simulink model "force_control"  (R2021b)
settings: Solver=FixedStepAuto  StartTime=0.0  StopTime=5  FixedStep=Ts  RelTol=1e-3
undefined symbols (not defined in the file): dqi, fd, invMd, K, KD, KF, KI, KP, Md, myRobot, qf, qi, qr, xr
libraries: vrlib x1
settings Model: Creator=simon  LastModifiedBy=luigi
settings SolverCC: ZeroCrossControl=DisableAll  AlgebraicLoopSolver=TrustRegion
settings DebuggingCC: SFMachineParentedDataDiag=warning

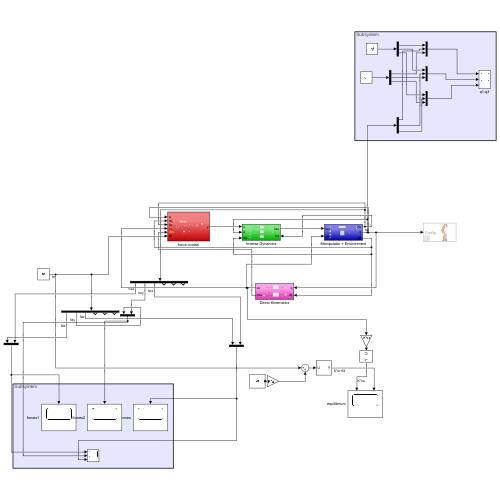
[thumbnail: Simulink's stored preview of the top-level diagram]
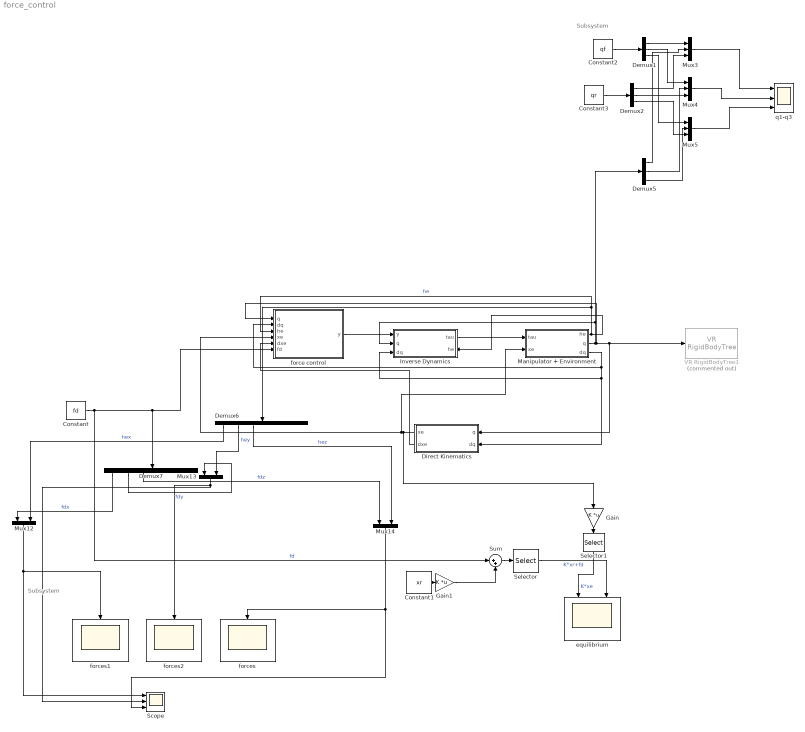
== system force_control ==
  note: Subsystem
  note: Subsystem
  Constant : Constant  Value=fd
  Constant1 : Constant  Value=xr
  Constant2 : Constant  Value=qf
  Constant3 : Constant  Value=qr
  Demux1 : Demux  Outputs=3
  Demux2 : Demux  Outputs=3
  Demux5 : Demux  Outputs=myRobot.N
  Demux6 : Demux  Outputs=6
  Demux7 : Demux  Outputs=6
  Direct Kinematics : Subsystem
  Gain : Gain  Gain=K  Multiplication=Matrix(K*u)
  Gain1 : Gain  Gain=K  Multiplication=Matrix(K*u)
  Inverse Dynamics : Subsystem
      settings: PortSchema="{\"entries\":[{\"content\":{\"sides\":[{\"content\":{\"connectorIds\":[\"In1\",\"In2\",\"In3\"]},\"type\":\"ConnectorPlacement.EquallySpacedRectSide\",\"uuid\":\"75fd2aef-6636-4229-8361-fd4aaeafc71d\"},{\"content\":{\"connectorIds\":[\"Out1\",\"In4\"],\"side\":\"RIGHT\"},\"type\":\"ConnectorPlacement.EquallySpacedRectSide\",\"uuid\":\"1144ef1f-b296-4ded-9ece-76b41f9ae70a\"},{\"content\":{\"connectorIds\":[],\"side\":\"TOP\"},\"type\":\"ConnectorPlacement.EquallySpacedRectSide\",\"uuid\":\"a2369661-a37d-42fa-931f-950a2098898d\"},{\"content\":{\"connectorIds\":[],\"side\":\"BOTTOM\"},\"type\":\"ConnectorPlacement.EquallySpacedRectSide\",\"uuid\":\"99474d0a-a266-4b98-966c-e86b0204795e\"},{\"content\":{\"connectorIds\":[],\"side\":\"HIDDEN\"},\"type\":\"ConnectorPlacement.EquallySpacedRectSide\",\"uuid\":\"b2ea56db-8612-481b-8b10-64691d881ee0\"}]},\"type\":\"ConnectorPlacement.EquallySpacedConnector\",\"uuid\":\"7eb160dc-bfe8-4791-8ee2-e581093abb5e\"}],\"packageUris\":[\"http://schema.mathworks.com/mf0/Connector/R2020b\"],\"version\":\"1.0\"}"
  Manipulator + Environment : Subsystem
  Mux12 : Mux  Inputs=2
  Mux13 : Mux  Inputs=2
  Mux14 : Mux  Inputs=2
  Mux3 : Mux  Inputs=3
  Mux4 : Mux  Inputs=3
  Mux5 : Mux  Inputs=3
  Scope : Scope  NumInputPorts=3
  Selector : Selector  InputPortWidth=6  IndexOptions=Index vector (dialog)  Indices=3  OutputSizes=1
  Selector1 : Selector  InputPortWidth=6  IndexOptions=Index vector (dialog)  Indices=3  OutputSizes=1
  Sum : Sum  Inputs=|++
  VR RigidBodyTree1 : vrlib/VR RigidBodyTree  Commented=on  RBT=rbt  useRBT=on  Ts=-1  ForceViewerOpen=on
      settings: SourceProductBaseCode=SL
  equilibrium : Scope  NumInputPorts=2
  force control : Subsystem
  forces : Scope
  forces1 : Scope
  forces2 : Scope
  q1-q3 : Scope  NumInputPorts=3
  wires:
  Direct Kinematics/2(dxe) -> force control/5(dxe)
  force control/1(y) -> Inverse Dynamics/1(y)
  Inverse Dynamics/1(tau) -> Manipulator + Environment/1(tau)
  Manipulator + Environment/3(dq) -> Inverse Dynamics/3(dq), Direct Kinematics/2(dq), force control/2(dq)
  Manipulator + Environment/1(he) -> Demux6/1, force control/3(he), Inverse Dynamics/4(he)  "he"
  Demux7/3 -> Mux14/1  "fdz"
  Direct Kinematics/1(xe) -> Manipulator + Environment/2(xe), force control/4(xe), Gain/1
  Constant/1 -> force control/6(fd), Demux7/1, Sum/1  "fd"
  Demux7/2 -> Mux13/1  "fdy"
  Demux7/1 -> Mux12/1  "fdx"
  Demux6/2 -> Mux13/2  "hey"
  Demux6/1 -> Mux12/2  "hex"
  Demux6/3 -> Mux14/2  "hez"
  Constant1/1 -> Gain1/1
  Selector1/1 -> equilibrium/1  "K*xe"
  Gain/1 -> Selector1/1
  Gain1/1 -> Sum/2
  Sum/1 -> Selector/1
  Selector/1 -> equilibrium/2  "K*xr+fd"
  Mux13/1 -> Scope/2, forces2/1
  Mux14/1 -> Scope/3, forces/1
  Mux12/1 -> Scope/1, forces1/1
  Manipulator + Environment/2(q) -> VR RigidBodyTree1/1, Direct Kinematics/1(q), force control/1(q), Demux5/1, Inverse Dynamics/2(q)
  Demux2/3 -> Mux5/3
  Constant3/1 -> Demux2/1
  Demux2/1 -> Mux3/3
  Demux2/2 -> Mux4/3
  Mux4/1 -> q1-q3/2
  Constant2/1 -> Demux1/1
  Demux1/3 -> Mux5/1
  Mux3/1 -> q1-q3/1
  Demux5/2 -> Mux4/2
  Demux5/3 -> Mux5/2
  Mux5/1 -> q1-q3/3
  Demux5/1 -> Mux3/2
  Demux1/2 -> Mux4/1
  Demux1/1 -> Mux3/1

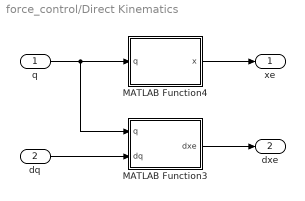
== system force_control/Direct Kinematics ==
  q : Inport
  dq : Inport  Port=2
  MATLAB Function3 : MATLAB Function  TreatAsAtomicUnit=on
  MATLAB Function4 : MATLAB Function  TreatAsAtomicUnit=on
  xe : Outport
  dxe : Outport  Port=2
  wires:
  MATLAB Function3/1(dxe) -> dxe/1
  dq/1 -> MATLAB Function3/2(dq)
  q/1 -> MATLAB Function3/1(q), MATLAB Function4/1(q)
  MATLAB Function4/1(x) -> xe/1

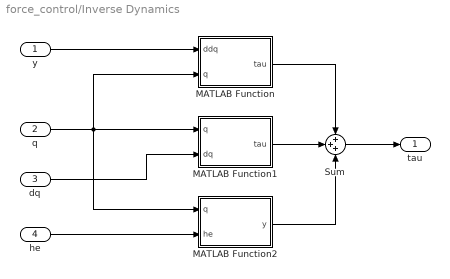
== system force_control/Inverse Dynamics ==
  y : Inport
  q : Inport  Port=2
  dq : Inport  Port=3
  he : Inport  Port=4
  MATLAB Function : MATLAB Function  TreatAsAtomicUnit=on
  MATLAB Function1 : MATLAB Function  TreatAsAtomicUnit=on
  MATLAB Function2 : MATLAB Function  TreatAsAtomicUnit=on
  Sum : Sum  Inputs=+++
  tau : Outport
  wires:
  MATLAB Function1/1(tau) -> Sum/2
  MATLAB Function/1(tau) -> Sum/1
  y/1 -> MATLAB Function/1(ddq)
  Sum/1 -> tau/1
  dq/1 -> MATLAB Function1/2(dq)
  q/1 -> MATLAB Function1/1(q), MATLAB Function2/1(q), MATLAB Function/2(q)
  he/1 -> MATLAB Function2/2(he)
  MATLAB Function2/1(y) -> Sum/3

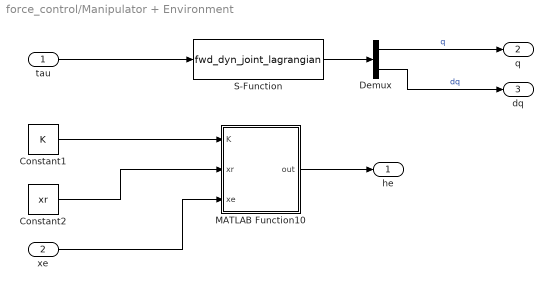
== system force_control/Manipulator + Environment ==
  tau : Inport
  xe : Inport  Port=2
  Constant1 : Constant  Value=K
  Constant2 : Constant  Value=xr
  Demux : Demux  Outputs=2
  MATLAB Function10 : MATLAB Function  TreatAsAtomicUnit=on
  S-Function : S-Function  FunctionName=fwd_dyn_joint_lagrangian  Parameters=myRobot,qi,dqi  SFunctionDeploymentMode=off  EnableBusSupport=off
  he : Outport
  q : Outport  Port=2
  dq : Outport  Port=3
  wires:
  tau/1 -> S-Function/1
  Constant1/1 -> MATLAB Function10/1(K)
  Constant2/1 -> MATLAB Function10/2(xr)
  xe/1 -> MATLAB Function10/3(xe)
  S-Function/1 -> Demux/1
  Demux/1 -> q/1  "q"
  Demux/2 -> dq/1  "dq"
  MATLAB Function10/1(out) -> he/1

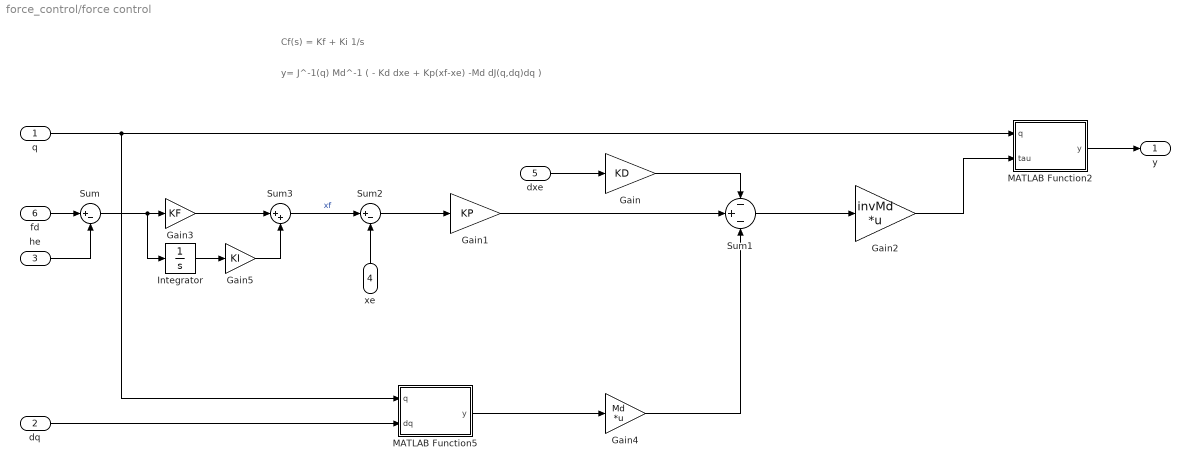
== system force_control/force control ==
  note: Cf(s) = Kf + Ki 1/s
  note: y= J^-1(q) Md^-1 ( - Kd dxe + Kp(xf-xe) -Md dJ(q,dq)dq )
  q : Inport
  dq : Inport  Port=2
  he : Inport  Port=3
  xe : Inport  Port=4
  dxe : Inport  Port=5
  fd : Inport  Port=6
  Gain : Gain  Gain=KD
  Gain1 : Gain  Gain=KP
  Gain2 : Gain  Gain=invMd  Multiplication=Matrix(K*u)
  Gain3 : Gain  Gain=KF
  Gain4 : Gain  Gain=Md  Multiplication=Matrix(K*u)
  Gain5 : Gain  Gain=KI
  Integrator : Integrator
  MATLAB Function2 : MATLAB Function  TreatAsAtomicUnit=on
  MATLAB Function5 : MATLAB Function  TreatAsAtomicUnit=on
  Sum : Sum  Inputs=|+-
  Sum1 : Sum  Inputs=-+-
  Sum2 : Sum  Inputs=|+-
  Sum3 : Sum  Inputs=|++
  y : Outport
  wires:
  MATLAB Function5/1(y) -> Gain4/1
  Gain2/1 -> MATLAB Function2/2(tau)
  MATLAB Function2/1(y) -> y/1
  dxe/1 -> Gain/1
  Sum1/1 -> Gain2/1
  Sum2/1 -> Gain1/1
  q/1 -> MATLAB Function5/1(q), MATLAB Function2/1(q)
  dq/1 -> MATLAB Function5/2(dq)
  Gain/1 -> Sum1/1
  xe/1 -> Sum2/2
  Gain1/1 -> Sum1/2
  Gain4/1 -> Sum1/3
  fd/1 -> Sum/1
  Sum/1 -> Integrator/1, Gain3/1
  he/1 -> Sum/2
  Integrator/1 -> Gain5/1
  Gain3/1 -> Sum3/1
  Gain5/1 -> Sum3/2
  Sum3/1 -> Sum2/1  "xf"

== matlab function force_control/Inverse Dynamics/MATLAB Function2 ==
  data: q input; he input; y output
function y = fcn(q, he)
y = getJ(q)'*he;

== matlab function force_control/force control/MATLAB Function5 ==
  data: q input; y output; dq input
function y = dJa(q, dq)

y = getDiffJa(q,dq)*dq;

== matlab function force_control/Direct Kinematics/MATLAB Function3 ==
  data: q input; dxe output; dq input
function dxe = Ja(q, dq)

dxe = getJa(q)*dq;

== matlab function force_control/force control/MATLAB Function2 ==
  data: q input; y output; tau input
function y = invJ(q, tau)

y = getInvJ(q)*tau;

== matlab function force_control/Direct Kinematics/MATLAB Function4 ==
  data: q input; x output
function x = k(q)

x = getK(q);

== matlab function force_control/Inverse Dynamics/MATLAB Function ==
  data: ddq input size=3; q input size=3; tau output
function tau = B(ddq, q)

tau = getB(q)*ddq;

== matlab function force_control/Inverse Dynamics/MATLAB Function1 ==
  data: q input size=3; tau output; dq input size=3
function tau = n(q, dq)

tau = getN(q, dq);

== matlab function force_control/Manipulator + Environment/MATLAB Function10 ==
  data: K input; out output size=6; xr input; xe input size=6
function out = hde(K,xr, xe)
%consider the interaction only in z direction
if xe(3) < xr(3)
    out = K*(xe-xr);
else 
    out = zeros(6,1);
end
